simulink model "X_position_CL"  (R2022b)
settings: Solver=FixedStepAuto  StartTime=0.0  StopTime=inf  FixedStep=0.043  RelTol=1e-3
undefined symbols (not defined in the file): Angular, Linear
libraries: robotlib x3
settings Model: Creator=yoav  LastModifiedBy=yoav
settings SolverCC: InsertRTBMode=Never (minimum delay)
settings OptimizationCC: EnhancedBackFolding=on  PassReuseOutputArgsAs=Individual arguments  ZeroExternalMemoryAtStartup=off  ZeroInternalMemoryAtStartup=off  MaxStackSize=64  OptimizeBlockOrder=speed  DifferentSizesBufferReuse=on  OptimizationCustomize=off  EfficientTunableParamExpr=on
settings DebuggingCC: ParameterTunabilityLossMsg=error
settings HardwareCC: ProdBitPerPointer=32  ProdBitPerSizeT=32  ProdBitPerPtrDiffT=32  ProdLargestAtomicFloat=None  ProdIntDivRoundTo=Undefined  ProdEndianess=Unspecified  ProdWordSize=32  ProdHWDeviceType=Generic->Unspecified (assume 32-bit Generic)
settings SFSimCC: MATLABDynamicMemAlloc=off
settings RTWCC: Description=Embedded Coder  SystemTargetFile=ert.tlc  HardwareBoard=Robot Operating System (ROS)  TLCOptions="-aInlineSetEventsForThisBaseRateFcn=TLC_FALSE -aSuppressMultiTaskScheduler=TLC_FALSE  -aRateBasedStepFcn=0"  TemplateMakefile=ert_default_tmf  Toolchain=Catkin  TargetLang=C++
settings CodeAppCC: ForceParamTrailComments=on  IgnoreCustomStorageClasses=off  OperatorAnnotations=on  SimulinkDataObjDesc=on  SFDataObjDesc=on  InsertBlockDesc=on
settings ERTTargetCC: ExtMode=on  ExtModeMexArgs='192.168.1.155' 0 17725

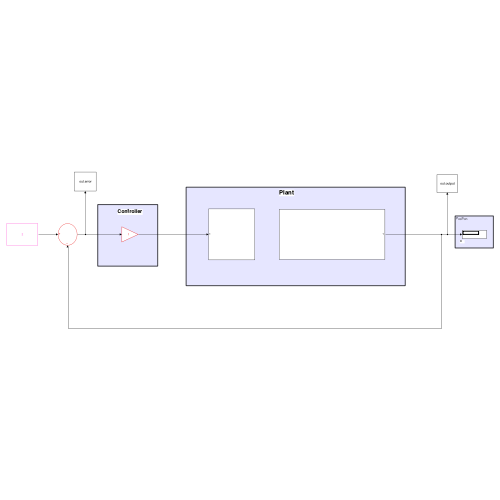
[thumbnail: Simulink's stored preview of the top-level diagram]
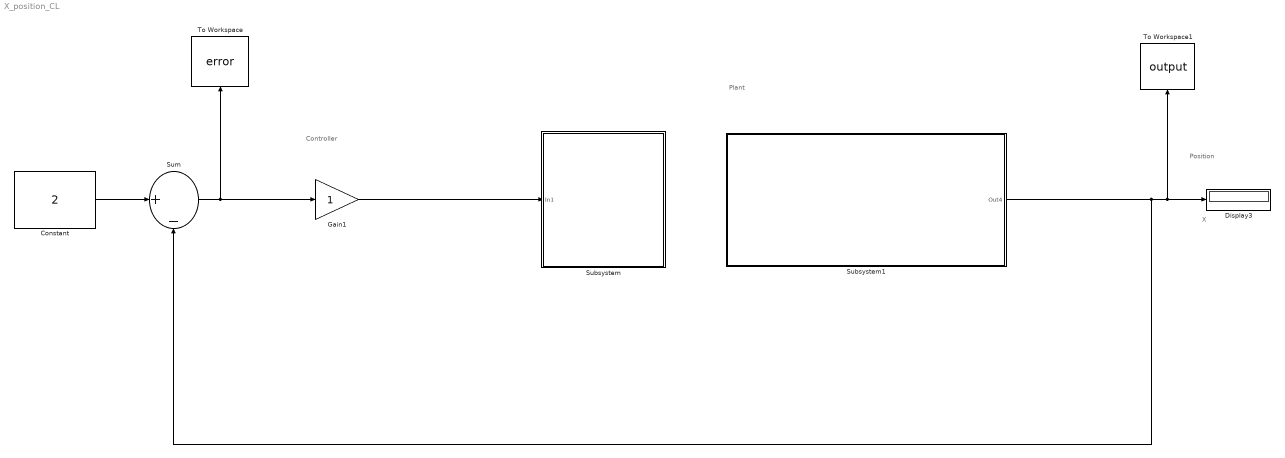
== system X_position_CL ==
  note: Controller
  note: Plant
  note: Position
  note: X
  Constant : Constant  Value=2
  Display3 : Display
  Gain1 : Gain
  Subsystem : Subsystem
  Subsystem1 : Subsystem
  Sum : Sum  Inputs=|+-
  To Workspace : ToWorkspace  VariableName=error  SaveFormat=Timeseries  SampleTime=-1
  To Workspace1 : ToWorkspace  VariableName=output  SaveFormat=Timeseries  SampleTime=-1
  wires:
  Subsystem1/1(Out4) -> Sum/2, Display3/1, To Workspace1/1
  Constant/1 -> Sum/1
  Sum/1 -> To Workspace/1, Gain1/1
  Gain1/1 -> Subsystem/1(In1)

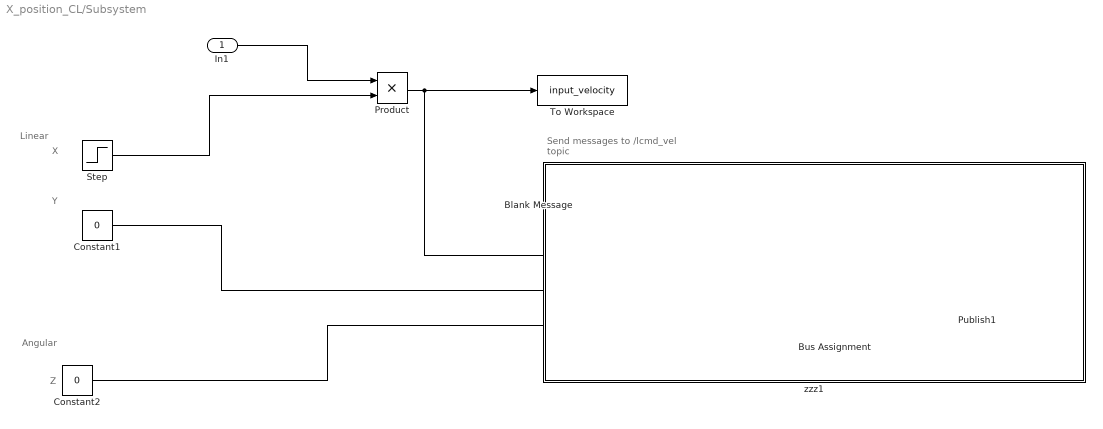
== system X_position_CL/Subsystem ==
  note: Send messages to /lcmd_vel topic
  note: Y
  note: X
  note: Linear
  note: Angular
  note: Z
  In1 : Inport
  Blank Message : robotlib/Blank Message  messageClass=Message  entityType=geometry_msgs/Twist  messageType=geometry_msgs/Twist  SampleTime=inf  legacyBusStruct=off
  Bus Assignment : BusAssignment  AssignedSignals=Linear.X,Linear.Y,Angular.Z
  Constant1 : Constant  Value=0
  Constant2 : Constant  Value=0
  Product : Product
  Publish1 : robotlib/Publish  topicSource=Specify your own  topic=/cmd_vel  messageType=geometry_msgs/Twist  legacyBusStruct=off  messageQueueLength=105
  Step : Step  Time=0  SampleTime=0
  To Workspace : ToWorkspace  VariableName=input_velocity  SaveFormat=Timeseries  SampleTime=-1
  zzz1 : Subsystem  TreatAsAtomicUnit=on
      settings: OpenFcn=% no-op
      mask Display: disp('')
  wires:
  Blank Message/1 -> Bus Assignment/1
  Bus Assignment/1 -> Publish1/1
  Constant2/1 -> Bus Assignment/4
  Constant1/1 -> Bus Assignment/3
  In1/1 -> Product/1
  Step/1 -> Product/2
  Product/1 -> Bus Assignment/2, To Workspace/1

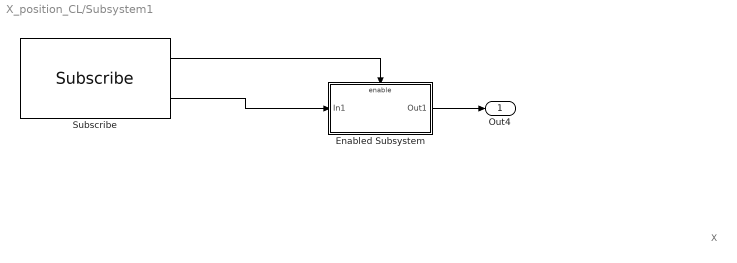
== system X_position_CL/Subsystem1 ==
  note: X
  Enabled Subsystem : Subsystem  TreatAsAtomicUnit=on
  Subscribe : robotlib/Subscribe  topicSource=Select from ROS network  topic=/odom  messageType=nav_msgs/Odometry  SampleTime=-1  legacyBusStruct=off  messageQueueLength=1
      settings: LibrarySourceBlock=roslib/ROS/Subscribe
  Out4 : Outport
  wires:
  Subscribe/2 -> Enabled Subsystem/1(In1)
  Subscribe/1 -> Enabled Subsystem/Enable
  Enabled Subsystem/1(Out1) -> Out4/1

== system X_position_CL/Subsystem/zzz1 ==

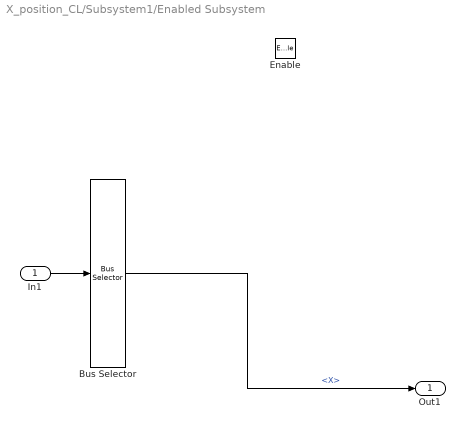
== system X_position_CL/Subsystem1/Enabled Subsystem ==
  In1 : Inport
  Enable : EnablePort
  Bus Selector : BusSelector  OutputSignals=Pose.Pose.Position.X
  Out1 : Outport
  wires:
  In1/1 -> Bus Selector/1
  Bus Selector/1 -> Out1/1  "<X>"
